simulink model "DiscreteControllerOnly"  (Simulink 8.1)
settings: Solver=ode45  StartTime=0.0  StopTime=10.0  RelTol=1e-3
settings Model: Creator=root  LastModifiedBy=root
settings DataIOCC: SignalLoggingSaveFormat=Dataset
settings OptimizationCC: ExpressionDepthLimit=128
settings DebuggingCC: FcnCallInpInsideContextMsg=EnableAllAsError
settings GRTTargetCC: CombineOutputUpdateFcns=on  GRTInterface=off

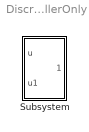
== system DiscreteControllerOnly ==
  Subsystem : Subsystem

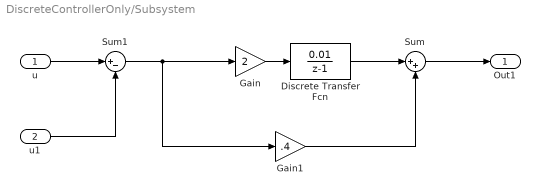
== system DiscreteControllerOnly/Subsystem ==
  u : Inport  OutDataTypeStr=double
  u1 : Inport  Port=2  OutDataTypeStr=double
  Discrete Transfer Fcn : DiscreteTransferFcn  Numerator=[0.01]  Denominator=[1 -1]  SampleTime=0.01
  Gain : Gain  Gain=2
  Gain1 : Gain  Gain=.4
  Sum : Sum  Inputs=|++
  Sum1 : Sum  Inputs=|+-
  Out1 : Outport  OutDataTypeStr=double
  wires:
  Sum1/1 -> Gain1/1, Gain/1
  Sum/1 -> Out1/1
  Gain1/1 -> Sum/2
  Discrete Transfer Fcn/1 -> Sum/1
  Gain/1 -> Discrete Transfer Fcn/1
  u/1 -> Sum1/1
  u1/1 -> Sum1/2
